simulink model "APF_SoftLanding_Quadrotor"  (R2023a)
settings: Solver=VariableStepAuto  StartTime=0.0  StopTime=120  RelTol=1e-3
values from neighbouring files (symbols this model uses):
  alpha_t = pi/2    (= 1.57079632679)    [Parameters.m]
  d0 = 7    [Parameters.m]
  k1 = 0.1395    [Parameters.m]
  k2 = 0.1784    [Parameters.m]
  k3 = 0.0442    [Parameters.m]
  ka = 0.2    [Parameters.m]
  katt = 10    [Parameters.m]
  kb = 0.6    [Parameters.m]
  kc = 0.4    [Parameters.m]
  krep = 90000    [Parameters.m]
  m = 5    [Parameters.m]
  maxRange = 10    [Parameters.m]
  n = 3    [Parameters.m]
  P_psi_lead = 2    [Parameters.m]
  P_vel_lead = 5    [Parameters.m]
  posHpad = [-25 -25 0]    [Parameters.m]
  Rmin = 0.1    [Parameters.m]
  target = [-25 -25 -5]    [Parameters.m]
  theta_des = pi/4    (= 0.785398163397)    [Parameters.m]
  thresholdLanding = 15    [Parameters.m]
  v_max = 2    [Parameters.m]
  zeta_des = 0    [Parameters.m]
  zGround = -0.15    [Parameters.m]
undefined symbols (not defined in the file or in its folder): Lidar, numobs, obs, platformUAV
libraries: uavsimlib x5, sharedtransform x2, uavalgslib x1, uavutilslib x1
(part 2 of 3)

== matlab function APF_SoftLanding_Quadrotor/MATLAB Function ==
function [V_cmd, yaw_cmd, Stop] = APF_Planner(pos, goal, obs, katt, krep, d0, v_max, numobs)

% =========================================================
% APF Planner for 3D Quadrotor
% pos  : [1x3] UAV position [N E D]
% goal : [1x3] goal position [N E D]
% obs  : [1x3] obstacle position [N E D]
% V_cmd: [1x3] velocity command [VN VE VD]
% =========================================================

% ---------------------------------------------------------
% 1. Initialize outputs with FIXED SIZE
% ---------------------------------------------------------

V_cmd   = zeros(1,3);
yaw_cmd = 0.0;
Stop    = 0.0;
F_att = zeros(1,3);
F_total = zeros(1,3);



% ---------------------------------------------------------
% 2. Force inputs to fixed-size row vectors
% ---------------------------------------------------------

p = zeros(1,3);
g = zeros(1,3);

p(1) = pos(1);
p(2) = pos(2);
p(3) = pos(3);

g(1) = goal(1);
g(2) = goal(2);
g(3) = goal(3);


% Scalar
v_lim = v_max(1);

% Khoảng cách từ UAV đến target
d_goal = g - p;
d_goal_mag = sqrt(d_goal(1)^2 + d_goal(2)^2 + d_goal(3)^2);

% ---------------------------------------------------------
% 3. Attractive force
% ---------------------------------------------------------

    F_att(1) = 2 * katt * d_goal(1);
    F_att(2) = 2 * katt * d_goal(2);
    F_att(3) = 2 * katt * d_goal(3);

% ---------------------------------------------------------
% 4. Repulsive force
% ---------------------------------------------------------



% ---------------------------------------------------------
% 5. Total force
% ---------------------------------------------------------

F_total(1) = F_att(1); 
F_total(2) = F_att(2);
F_total(3) = F_att(3);

F_norm = sqrt(F_total(1)^2 + F_total(2)^2 + F_total(3)^2);


% ---------------------------------------------------------
% 6. Generate velocity command
% ---------------------------------------------------------

if d_goal_mag < 0.15

    V_cmd(1,1) = 0;
    V_cmd(1,2) = 0;
    V_cmd(1,3) = 0;

    Stop = 1.0;

elseif F_norm > 1e-4

    V_cmd(1) = v_lim * F_total(1) / F_norm;
    V_cmd(2) = v_lim * F_total(2) / F_norm;
    V_cmd(3) = v_lim * F_total(3) / F_norm;

else

    V_cmd(1) = 0;
    V_cmd(2) = 0;
    V_cmd(3) = 0;

end

% ---------------------------------------------------------
% 7. Yaw command
% ---------------------------------------------------------

V_horizontal = sqrt(V_cmd(1)^2 + V_cmd(2)^2);

if V_horizontal > 0.05

    yaw_cmd = atan2(V_cmd(2), V_cmd(1));

else

    yaw_cmd = 0.0;

end

end


%% =========================================================================
%% =========================================================================

% function [V_cmd, yaw_cmd, Stop] = APF_Planner(pos, goal, obs, katt, krep, d0, v_max, numobs)
% 
% % =========================================================
% % Improved APF Planner for 3D UAV
% %
% % Coordinate frame: NED
% %
% % FEATURES
% %   1. Attractive force
% %   2. Improved repulsive force for GNRON
% %   3. Local-minimum detection
% %   4. Dynamic tangent escape
% %   5. Forward-looking tangent selection
% %   6. Directional weighting for oscillation suppression
% %   7. Speed scheduling
% %
% % INPUTS
% %   pos     : UAV position        [1x3] [N E D]
% %   goal    : Goal position       [1x3] [N E D]
% %   obs     : Obstacle positions  [Nx3] [N E D]
% %   katt    : Attractive gain
% %   krep    : Repulsive gain
% %   d0      : Obstacle influence distance [m]
% %   v_max   : Maximum velocity [m/s]
% %   numobs  : Number of obstacles
% %
% % OUTPUTS
% %   V_cmd   : Velocity command [1x3] [VN VE VD]
% %   yaw_cmd : Heading command [rad]
% %   Stop    : 1 when goal reached
% %
% % =========================================================
% 
% 
% %% ========================================================
% % 1. INITIALIZATION
% % =========================================================
% 
% V_cmd   = zeros(1,3);
% yaw_cmd = 0.0;
% Stop    = 0.0;
% 
% F_att     = zeros(1,3);
% F_rep     = zeros(1,3);
% F_cmd_raw = zeros(1,3);
% 
% p = zeros(1,3);
% g = zeros(1,3);
% 
% p(1) = pos(1);
% p(2) = pos(2);
% p(3) = pos(3);
% 
% g(1) = goal(1);
% g(2) = goal(2);
% g(3) = goal(3);
% 
% % Đại lượng tránh chia cho 0 
% small_num = 1e-6;
% 
% 
% %% ========================================================
% % 2. PARAMETERS
% % =========================================================
% 
% % Ngưỡng xác định UAV đã tới goal.
% goal_tol = 0.30;          % [m]
% 
% % ---------------------------------------------------------
% % Local minimum detection
% % ---------------------------------------------------------
% 
% % Nếu F_total < F_enter --> Local Minima --> Bật Tangent
% F_enter = 0.10;
% 
% % Nếu F_total > F_exit --> Thoát khỏi Local Minima
% % F_enter < F_total < F_exit --> Vẫn bật Tangent, F_enter < F_exit để tránh Tangent bật tắt liên tục 
% F_exit  = 0.30;
% 
% % Khoảng cách giữa UAV và target phải lớn hơn goal_min_dist thì mới được
% % coi là Local Minima
% goal_min_dist = 0.50;
% 
% 
% % ---------------------------------------------------------
% % Tangential force
% % ---------------------------------------------------------
% 
% % Hệ số độ mạnh của lực tiếp tuyến
% k_tan = 1.0;
% 
% % Number of directions searched on tangent plane (Mặt phẳng tiếp tuyến
% % vuông góc với vector hướng từ Obs ra UAV
% N_tangent = 12;
% 
% % Prediction horizon for tangent evaluation
% N_pred = 3;
% 
% % Prediction distance (Xem UAV sẽ ở đâu)
% look_ahead = 0.25*d0;
% 
% if look_ahead < 0.30
%     look_ahead = 0.30;
% end
% 
% 
% % Tangent candidate cost
% w_goal  = 1.0;
% w_clear = 1.0;
% w_prev  = 0.60;
% 
% 
% % ---------------------------------------------------------
% % Oscillation suppression
% %
% % Δalpha <= pi/6:
% %       m = m'
% %
% % pi/6 < Δalpha <= pi/3:
% %       m > m'
% %
% % Δalpha > pi/3:
% %       m >> m'
% %
% % Numerical values below are implementation choices.
% % ---------------------------------------------------------
% 
% theta_small = pi/6;
% theta_large = pi/3;
% 
% % Small direction change
% m_prev_1 = 0.50;
% m_new_1  = 0.50;
% 
% % Medium direction change
% m_prev_2 = 0.70;
% m_new_2  = 0.30;
% 
% % Large direction change
% m_prev_3 = 0.90;
% m_new_3  = 0.10;
% 
% 
% %% ========================================================
% % 3. PERSISTENT STATES
% % =========================================================
% 
% persistent tangent_active
% persistent tangent_prev
% persistent previous_obs_idx
% 
% persistent prev_move_dir
% persistent prev_dir_valid
% 
% 
% if isempty(tangent_active)
%     tangent_active = false;
% end
% 
% if isempty(tangent_prev)
%     tangent_prev = zeros(1,3);
% end
% 
% if isempty(previous_obs_idx)
%     previous_obs_idx = 0;
% end
% 
% if isempty(prev_move_dir)
%     prev_move_dir = zeros(1,3);
% end
% 
% if isempty(prev_dir_valid)
%     prev_dir_valid = false;
% end
% 
% 
% %% ========================================================
% % 4. NUMBER OF OBSTACLES
% % =========================================================
% 
% Nobs = numobs;
% 
% if Nobs > size(obs,1)
%     Nobs = size(obs,1);
% end
% 
% if Nobs < 0
%     Nobs = 0;
% end
% 
% 
% %% ========================================================
% % 5. GOAL VECTOR
% % =========================================================
% 
% goal_vec = g - p;
% 
% d_goal = sqrt(goal_vec(1)^2 + goal_vec(2)^2 + goal_vec(3)^2);
% 
% 
% %% ========================================================
% % 6. GOAL REACHED
% % =========================================================
% 
% if d_goal <= goal_tol
% 
%     V_cmd   = zeros(1,3);
%     yaw_cmd = 0.0;
%     Stop    = 1.0;
% 
%     % Reset memory
%     tangent_active   = false;
%     tangent_prev     = zeros(1,3);
%     previous_obs_idx = 0;
% 
%     prev_move_dir = zeros(1,3);
%     prev_dir_valid = false;
% 
%     return;
% end
% 
% 
% dir_goal = goal_vec / max(d_goal,small_num);
% 
% 
% %% ========================================================
% % 7. ATTRACTIVE FORCE
% % =========================================================
% %
% % Uatt = katt*d_goal^2
% %
% % Fatt = 2*katt*(goal-pos)
% %
% 
% F_att = 2.0*katt*goal_vec;
% 
% 
% %% ========================================================
% % 8. IMPROVED REPULSIVE FORCE
% %
% % GNRON improvement
% %
% % Frep = Frep1 + Frep2
% % =========================================================
% 
% min_obs_dist = 1e6;
% nearest_idx  = 0;
% 
% 
% for i = 1:Nobs
% 
%     obs_i = zeros(1,3);
% 
%     obs_i(1) = obs(i,1);
%     obs_i(2) = obs(i,2);
%     obs_i(3) = obs(i,3);
% 
% 
%     % Vector obstacle -> UAV
%     obs_vec = p - obs_i;
% 
%     d_obs = sqrt(obs_vec(1)^2 + obs_vec(2)^2 + obs_vec(3)^2);
% 
% 
%     % Nearest obstacle
%     if d_obs < min_obs_dist
%         min_obs_dist = d_obs;
%         nearest_idx  = i;
%     end
% 
% 
%     if d_obs <= d0
% 
%         d_safe = max(d_obs,small_num);
% 
%         dir_away = obs_vec/d_safe;
% 
% 
%         % -------------------------------------------------
%         % Goal-distance weighting
%         %
%         % Approaches zero when UAV approaches goal
%         % -------------------------------------------------
% 
%         exp_goal = exp(-d_goal);
% 
%         weight_rep = 1.0/(1.0 + exp_goal) - 0.5;
% 
% 
%         % -------------------------------------------------
%         % Frep1
%         % -------------------------------------------------
% 
%         coeff1 = 2.0 * krep * (1.0/d_safe - 1.0/d0) * (1.0/(d_safe^2)) * weight_rep;
% 
%         F_rep1 = coeff1 * dir_away;
% 
% 
%         % -------------------------------------------------
%         % Frep2
%         % -------------------------------------------------
% 
%         sigmoid_derivative = exp_goal/((1.0 + exp_goal)^2);
% 
%         coeff2 = krep * (1.0/d_safe - 1.0/d0)^2 * sigmoid_derivative;
% 
%         F_rep2 = coeff2 * dir_goal;
% 
% 
%         F_rep = F_rep + F_rep1 + F_rep2;
% 
%     end
% 
% end
% 
% 
% %% ========================================================
% % 9. NORMAL APF RESULTANT FORCE
% % =========================================================
% 
% F_total = F_att + F_rep;
% 
% F_total_norm = sqrt(F_total(1)^2 + F_total(2)^2 + F_total(3)^2);
% 
% 
% %% ========================================================
% % 10. OBSTACLE NEARBY
% % =========================================================
% 
% obstacle_near = false;
% 
% if (Nobs > 0) && (min_obs_dist < d0)
%     obstacle_near = true;
% end
% 
% 
% %% ========================================================
% % 11. LOCAL MINIMUM DETECTION WITH HYSTERESIS
% % =========================================================
% 
% if ~tangent_active
% 
%     if (F_total_norm < F_enter) && (d_goal > goal_min_dist) && obstacle_near
% 
%         tangent_active = true;
% 
% 
%         % Do not use tangent from unrelated obstacle
%         if nearest_idx ~= previous_obs_idx
%             tangent_prev = zeros(1,3);
%         end
% 
%         previous_obs_idx = nearest_idx;
%     end
% 
% else
% 
%     if (F_total_norm > F_exit) || (~obstacle_near) || (d_goal <= goal_min_dist)
% 
%         tangent_active = false;
% 
%     end
% 
% end
% 
% 
% %% ========================================================
% % 12. DYNAMIC TANGENT ESCAPE
% %
% % Tangent is ONLY added when local minimum is active.
% % =========================================================
% 
% if tangent_active && nearest_idx > 0
% 
%     %% ----------------------------------------------------
%     % 12.1 Nearest obstacle normal
%     % -----------------------------------------------------
% 
%     obs_near = zeros(1,3);
% 
%     obs_near(1) = obs(nearest_idx,1);
%     obs_near(2) = obs(nearest_idx,2);
%     obs_near(3) = obs(nearest_idx,3);
% 
% 
%     normal_vec = p - obs_near;
% 
%     normal_norm = sqrt(normal_vec(1)^2 + normal_vec(2)^2 + normal_vec(3)^2);
% 
% 
%     if normal_norm > small_num
%         n = normal_vec/normal_norm;
%     else
%         n = -dir_goal;
%     end
% 
% 
%     %% ----------------------------------------------------
%     % 12.2 Construct tangent plane basis
%     % -----------------------------------------------------
% 
%     abs_n = abs(n);
% 
%     [~,idx_ref] = min(abs_n);
% 
%     ref = zeros(1,3);
%     ref(idx_ref) = 1.0;
% 
% 
%     e1 = cross(n,ref);
% 
%     e1_norm = sqrt(e1(1)^2 + e1(2)^2 + e1(3)^2);
% 
%     e1 = e1/max(e1_norm,small_num);
% 
% 
%     e2 = cross(n,e1);
% 
%     e2_norm = sqrt(e2(1)^2 + e2(2)^2 + e2(3)^2);
% 
%     e2 = e2/max(e2_norm,small_num);
% 
% 
%     %% ----------------------------------------------------
%     % 12.3 Forward-looking tangent search
%     %
%     % Inspired by paper Eq. (12)-(13)
%     %
%     % Every candidate tangent is predicted several
%     % positions ahead and evaluated by:
%     %
%     %   goal direction
%     %   obstacle clearance
%     %   continuity with previous tangent
%     % -----------------------------------------------------
% 
%     best_score = -1e9;
%     best_tangent = zeros(1,3);
% 
% 
%     tangent_prev_norm = sqrt(tangent_prev(1)^2 + tangent_prev(2)^2 + tangent_prev(3)^2);
% 
% 
%     for k = 1:N_tangent
% 
%         theta = 2.0 * pi * (k-1)/N_tangent;
% 
% 
%         t_candidate = cos(theta) * e1 + sin(theta) * e2;
% 
% 
%         t_norm = sqrt(t_candidate(1)^2 + t_candidate(2)^2 + t_candidate(3)^2);
% 
%         t_candidate = t_candidate/max(t_norm,small_num);
% 
% 
%         % ---------------------------------------------
%         % Goal-direction score
%         % ---------------------------------------------
% 
%         goal_score = dot(t_candidate,dir_goal);
% 
% 
%         % ---------------------------------------------
%         % Previous tangent continuity score
%         % ---------------------------------------------
% 
%         prev_score = 0.0;
% 
%         if tangent_prev_norm > 1e-4
% 
%             prev_tangent_dir = tangent_prev/tangent_prev_norm;
% 
%             prev_score = dot(t_candidate,prev_tangent_dir);
% 
%         end
% 
% 
%         % ---------------------------------------------
%         % Forward-looking clearance
%         % ---------------------------------------------
% 
%         min_pred_dist = 1e6;
% 
% 
%         for h = 1:N_pred
% 
%             pred_ratio = h/N_pred;
% 
%             p_test = p + pred_ratio * look_ahead * t_candidate;
% 
% 
%             for j = 1:Nobs
% 
%                 test_vec = zeros(1,3);
% 
%                 test_vec(1) = p_test(1) - obs(j,1);
% 
%                 test_vec(2) = p_test(2) - obs(j,2);
% 
%                 test_vec(3) = p_test(3) - obs(j,3);
% 
% 
%                 test_dist = sqrt(test_vec(1)^2 + test_vec(2)^2 + test_vec(3)^2);
% 
% 
%                 if test_dist < min_pred_dist
%                     min_pred_dist = test_dist;
%                 end
% 
%             end
% 
%         end
% 
% 
%         clear_score = min_pred_dist/max(d0,small_num);
% 
% 
%         if clear_score > 2.0
%             clear_score = 2.0;
%         end
% 
% 
%         % ---------------------------------------------
%         % Comprehensive score
%         % ---------------------------------------------
% 
%         score = w_goal*goal_score + w_clear*clear_score + w_prev*prev_score;
% 
% 
%         if score > best_score
% 
%             best_score = score;
% 
%             best_tangent = t_candidate;
% 
%         end
% 
%     end
% 
% 
%     % Store tangent for next sample
%     tangent_prev = best_tangent;
% 
% 
%     % Tangential force
%     F_tan = k_tan*best_tangent;
% 
% 
%     % APF + tangent
%     F_cmd_raw = F_total + F_tan;
% 
% 
% else
% 
%     % Normal operation
%     F_cmd_raw = F_total;
% 
% end
% 
% 
% %% ========================================================
% % 13. RAW COMMAND DIRECTION
% % =========================================================
% 
% F_raw_norm = sqrt(F_cmd_raw(1)^2 + F_cmd_raw(2)^2 + F_cmd_raw(3)^2);
% 
% 
% if F_raw_norm > small_num
% 
%     w_new = F_cmd_raw/F_raw_norm;
% 
% else
% 
%     w_new = dir_goal;
% 
% end
% 
% 
% %% ========================================================
% % 14. OSCILLATION SUPPRESSION
% %
% % Based on Eq. (10)-(11) of the paper.
% %
% % Paper:
% %
% % X(n+1) =
% %   X(n) + L*(m*w_n + m'*w_(n+1))
% %
% % Our planner outputs velocity instead of waypoint,
% % therefore:
% %
% % w_cmd =
% %   normalize(m*w_prev + m'*w_new)
% %
% % =========================================================
% 
% move_dir = w_new;
% 
% 
% % Apply directional continuity mainly near obstacles.
% if obstacle_near && prev_dir_valid
% 
%     % -----------------------------------------------------
%     % Angle between previous and current directions
%     % -----------------------------------------------------
% 
%     cos_alpha = dot(prev_move_dir,w_new);
% 
% 
%     % Numerical clamp
%     if cos_alpha > 1.0
%         cos_alpha = 1.0;
%     elseif cos_alpha < -1.0
%         cos_alpha = -1.0;
%     end
% 
% 
%     delta_alpha = acos(cos_alpha);
% 
% 
%     % -----------------------------------------------------
%     % Direction weighting according to paper Eq. (11)
%     % -----------------------------------------------------
% 
%     if delta_alpha <= theta_small
% 
%         % m = m'
%         m_prev = m_prev_1;
%         m_new  = m_new_1;
% 
% 
%     elseif delta_alpha <= theta_large
% 
%         % m > m'
%         m_prev = m_prev_2;
%         m_new  = m_new_2;
% 
% 
%     else
% 
%         % m >> m'
%         m_prev = m_prev_3;
%         m_new  = m_new_3;
% 
%     end
% 
% 
%     % -----------------------------------------------------
%     % Eq. (10)-style weighted direction
%     % -----------------------------------------------------
% 
%     w_weighted = m_prev*prev_move_dir + m_new*w_new;
% 
% 
%     w_weighted_norm = sqrt(w_weighted(1)^2 + w_weighted(2)^2 + w_weighted(3)^2);
% 
% 
%     if w_weighted_norm > small_num
% 
%         move_dir = w_weighted/w_weighted_norm;
% 
%     else
% 
%         move_dir = w_new;
% 
%     end
% 
% end
% 
% 
% % ---------------------------------------------------------
% % Save actual direction used
% % ---------------------------------------------------------
% 
% prev_move_dir = move_dir;
% prev_dir_valid = true;
% 
% 
% %% ========================================================
% % 15. SPEED SCHEDULING
% % =========================================================
% 
% % Slow near goal
% goal_speed_factor = d_goal/max(d0,small_num);
% 
% 
% if goal_speed_factor > 1.0
%     goal_speed_factor = 1.0;
% elseif goal_speed_factor < 0.15
%     goal_speed_factor = 0.15;
% end
% 
% 
% % Slow near obstacles
% obs_speed_factor = 1.0;
% 
% 
% if obstacle_near
% 
%     obs_speed_factor = min_obs_dist/max(d0,small_num);
% 
% 
%     if obs_speed_factor < 0.25
%         obs_speed_factor = 0.25;
%     elseif obs_speed_factor > 1.0
%         obs_speed_factor = 1.0;
%     end
% 
% end
% 
% 
% v_cmd_mag = v_max * goal_speed_factor * obs_speed_factor;
% 
% 
% % Do not become too slow while escaping local minimum
% if tangent_active
% 
%     v_escape_min = 0.35*v_max;
% 
%     if v_cmd_mag < v_escape_min
%         v_cmd_mag = v_escape_min;
%     end
% 
% end
% 
% 
% %% ========================================================
% % 16. VELOCITY COMMAND
% % =========================================================
% 
% V_cmd = v_cmd_mag * move_dir;
% 
% 
% %% ========================================================
% % 17. YAW COMMAND
% % =========================================================
% 
% horizontal_speed = sqrt(V_cmd(1)^2 + V_cmd(2)^2);
% 
% 
% if horizontal_speed > small_num
% 
%     yaw_cmd = atan2(V_cmd(2),V_cmd(1));
% 
% else
% 
%     yaw_cmd = 0.0;
% 
% end
% 
% 
% Stop = 0.0;
% 
% end

%% ============================================================================
%% ===============================================================================

% function [V_cmd, yaw_cmd, Stop] = APF_Planner( ...
%     pos, goal, obs, katt, krep, d0, v_max, numobs)
% 
% % =========================================================
% % Improved APF Planner for 3D UAV
% %
% % Coordinate frame: NED
% %
% % Features:
% %   1. Attractive force
% %   2. Improved repulsive force for GNRON
% %   3. Local-minimum detection using resultant force
% %   4. Dynamic optimal tangential force
% %   5. Tangent hysteresis
% %   6. Tangent direction memory
% %   7. Speed scheduling
% %
% % INPUTS:
% %   pos     : UAV position        [1x3] [N E D]
% %   goal    : Goal position       [1x3] [N E D]
% %   obs     : Obstacle positions  [Nx3] [N E D]
% %   katt    : Attractive gain
% %   krep    : Repulsive gain
% %   d0      : Obstacle influence distance [m]
% %   v_max   : Maximum velocity [m/s]
% %   numobs  : Number of obstacles
% %
% % OUTPUTS:
% %   V_cmd   : Velocity command [1x3] [VN VE VD]
% %   yaw_cmd : Heading command [rad]
% %   Stop    : 1 when goal reached
% %
% % =========================================================
% 
% 
% %% ========================================================
% % 1. FIXED-SIZE INITIALIZATION
% % =========================================================
% 
% V_cmd   = zeros(1,3);
% yaw_cmd = 0.0;
% Stop    = 0.0;
% 
% F_att   = zeros(1,3);
% F_rep   = zeros(1,3);
% F_total = zeros(1,3);
% F_cmd   = zeros(1,3);
% 
% p = zeros(1,3);
% g = zeros(1,3);
% 
% p(1) = pos(1);
% p(2) = pos(2);
% p(3) = pos(3);
% 
% g(1) = goal(1);
% g(2) = goal(2);
% g(3) = goal(3);
% 
% small_num = 1e-6;
% 
% 
% %% ========================================================
% % 2. PARAMETERS
% % =========================================================
% 
% % Goal tolerance
% goal_tol = 0.30;          % [m]
% 
% % ---------------------------------------------------------
% % Local minimum detection
% % ---------------------------------------------------------
% %
% % Tangent is activated when:
% %
% %       |F_total| < F_enter
% %
% % and deactivated only when:
% %
% %       |F_total| > F_exit
% %
% % F_exit > F_enter creates hysteresis.
% %
% % IMPORTANT:
% % These values must be tuned according to katt/krep.
% % ---------------------------------------------------------
% 
% F_enter = 0.10;
% F_exit  = 0.30;
% 
% % UAV must still be sufficiently far from goal
% goal_min_dist = 0.50;     % [m]
% 
% 
% % ---------------------------------------------------------
% % Tangential force
% % ---------------------------------------------------------
% 
% k_tan = 1.0;
% 
% % Number of tangent candidate directions
% %
% % 12 -> every 30 degrees in tangent plane
% N_tangent = 12;
% 
% % Look-ahead distance used to evaluate tangent direction
% look_ahead = 0.25 * d0;
% 
% if look_ahead < 0.30
%     look_ahead = 0.30;
% end
% 
% % Cost-function weights
% w_goal  = 1.0;
% w_clear = 1.0;
% w_prev  = 0.6;
% 
% 
% %% ========================================================
% % 3. PERSISTENT STATES FOR TANGENT MODE
% % =========================================================
% 
% persistent tangent_active
% persistent tangent_prev
% persistent previous_obs_idx
% 
% if isempty(tangent_active)
%     tangent_active = false;
% end
% 
% if isempty(tangent_prev)
%     tangent_prev = zeros(1,3);
% end
% 
% if isempty(previous_obs_idx)
%     previous_obs_idx = 0;
% end
% 
% 
% %% ========================================================
% % 4. NUMBER OF OBSTACLES
% % =========================================================
% 
% Nobs = numobs;
% 
% if Nobs > size(obs,1)
%     Nobs = size(obs,1);
% end
% 
% if Nobs < 0
%     Nobs = 0;
% end
% 
% 
% %% ========================================================
% % 5. VECTOR TO GOAL
% % =========================================================
% 
% goal_vec = g - p;
% 
% d_goal = sqrt( ...
%     goal_vec(1)^2 + ...
%     goal_vec(2)^2 + ...
%     goal_vec(3)^2);
% 
% 
% %% ========================================================
% % 6. GOAL REACHED
% % =========================================================
% 
% if d_goal <= goal_tol
% 
%     V_cmd   = zeros(1,3);
%     yaw_cmd = 0.0;
%     Stop    = 1.0;
% 
%     % Reset tangent state
%     tangent_active   = false;
%     tangent_prev     = zeros(1,3);
%     previous_obs_idx = 0;
% 
%     return;
% 
% end
% 
% 
% % Unit vector toward goal
% dir_goal = goal_vec / max(d_goal, small_num);
% 
% 
% %% ========================================================
% % 7. ATTRACTIVE FORCE
% %
% % U_att = katt * d_goal^2
% %
% % F_att = 2*katt*(goal-pos)
% % =========================================================
% 
% F_att = 2.0 * katt * goal_vec;
% 
% 
% %% ========================================================
% % 8. IMPROVED REPULSIVE FORCE FOR GNRON
% % =========================================================
% 
% min_obs_dist = 1e6;
% nearest_idx  = 0;
% 
% 
% for i = 1:Nobs
% 
%     obs_i = zeros(1,3);
% 
%     obs_i(1) = obs(i,1);
%     obs_i(2) = obs(i,2);
%     obs_i(3) = obs(i,3);
% 
% 
%     % -----------------------------------------------------
%     % Vector from obstacle toward UAV
%     % -----------------------------------------------------
% 
%     obs_vec = p - obs_i;
% 
%     d_obs = sqrt( ...
%         obs_vec(1)^2 + ...
%         obs_vec(2)^2 + ...
%         obs_vec(3)^2);
% 
% 
%     % Find nearest obstacle
%     if d_obs < min_obs_dist
% 
%         min_obs_dist = d_obs;
%         nearest_idx  = i;
% 
%     end
% 
% 
%     % -----------------------------------------------------
%     % Only active inside obstacle influence distance
%     % -----------------------------------------------------
% 
%     if d_obs <= d0
% 
%         d_safe = max(d_obs, small_num);
% 
% 
%         % Unit direction away from obstacle
%         dir_away = obs_vec / d_safe;
% 
% 
%         % =================================================
%         % Goal-distance weighting
%         %
%         % Positive version of the weighting term is used
%         % here so that Frep1 points AWAY from obstacle.
%         %
%         % As d_goal -> 0:
%         %
%         % weight_rep -> 0
%         %
%         % therefore obstacle repulsion weakens near goal.
%         % =================================================
% 
%         exp_goal = exp(-d_goal);
% 
%         weight_rep = ...
%             1.0 / (1.0 + exp_goal) - 0.5;
% 
% 
%         % =================================================
%         % Frep1
%         % Main obstacle repulsive component
%         % =================================================
% 
%         coeff1 = ...
%             2.0 * krep ...
%             * (1.0/d_safe - 1.0/d0) ...
%             * (1.0/(d_safe^2)) ...
%             * weight_rep;
% 
%         F_rep1 = coeff1 * dir_away;
% 
% 
%         % =================================================
%         % Frep2
%         % Goal-oriented component
%         % =================================================
% 
%         sigmoid_derivative = ...
%             exp_goal / ((1.0 + exp_goal)^2);
% 
% 
%         coeff2 = ...
%             krep ...
%             * (1.0/d_safe - 1.0/d0)^2 ...
%             * sigmoid_derivative;
% 
% 
%         F_rep2 = coeff2 * dir_goal;
% 
% 
%         % =================================================
%         % Total obstacle contribution
%         % =================================================
% 
%         F_rep = F_rep + F_rep1 + F_rep2;
% 
%     end
% 
% end
% 
% 
% %% ========================================================
% % 9. NORMAL APF RESULTANT FORCE
% % =========================================================
% 
% F_total = F_att + F_rep;
% 
% F_norm = sqrt( ...
%     F_total(1)^2 + ...
%     F_total(2)^2 + ...
%     F_total(3)^2);
% 
% 
% %% ========================================================
% % 10. LOCAL MINIMUM / TANGENT ACTIVATION
% % =========================================================
% 
% % Tangent only allowed if an obstacle is actually nearby
% obstacle_near = false;
% 
% if (Nobs > 0) && (min_obs_dist < d0)
%     obstacle_near = true;
% end
% 
% 
% % ---------------------------------------------------------
% % Enter tangent mode
% % ---------------------------------------------------------
% 
% if ~tangent_active
% 
%     if (F_norm < F_enter) && ...
%        (d_goal > goal_min_dist) && ...
%        obstacle_near
% 
%         tangent_active = true;
% 
%         % New obstacle -> do not inherit tangent direction
%         % from an unrelated previous obstacle
%         if nearest_idx ~= previous_obs_idx
%             tangent_prev = zeros(1,3);
%         end
% 
%         previous_obs_idx = nearest_idx;
% 
%     end
% 
% else
% 
%     % -----------------------------------------------------
%     % Exit tangent mode
%     %
%     % Hysteresis:
%     %
%     % F_exit > F_enter
%     % -----------------------------------------------------
% 
%     if (F_norm > F_exit) || ...
%        (~obstacle_near) || ...
%        (d_goal <= goal_min_dist)
% 
%         tangent_active = false;
% 
%     end
% 
% end
% 
% 
% %% ========================================================
% % 11. DYNAMIC OPTIMAL TANGENT
% % =========================================================
% 
% if tangent_active && nearest_idx > 0
% 
%     % -----------------------------------------------------
%     % Nearest obstacle
%     % -----------------------------------------------------
% 
%     obs_near = zeros(1,3);
% 
%     obs_near(1) = obs(nearest_idx,1);
%     obs_near(2) = obs(nearest_idx,2);
%     obs_near(3) = obs(nearest_idx,3);
% 
% 
%     % -----------------------------------------------------
%     % Normal vector of obstacle surface
%     %
%     % n points:
%     %
%     % obstacle ---> UAV
%     % -----------------------------------------------------
% 
%     normal_vec = p - obs_near;
% 
%     normal_norm = sqrt( ...
%         normal_vec(1)^2 + ...
%         normal_vec(2)^2 + ...
%         normal_vec(3)^2);
% 
% 
%     if normal_norm > small_num
% 
%         n = normal_vec / normal_norm;
% 
%     else
% 
%         % Extremely unlikely case:
%         % UAV exactly at obstacle center
%         n = -dir_goal;
% 
%     end
% 
% 
%     % =====================================================
%     % 11.1 CREATE ORTHONORMAL BASIS ON TANGENT PLANE
%     %
%     % Choose reference axis least parallel to n.
%     %
%     % This axis is ONLY used to construct the tangent plane.
%     % Final tangent direction is optimized over 360 degrees.
%     % =====================================================
% 
%     abs_n = abs(n);
% 
%     [~, idx_ref] = min(abs_n);
% 
%     ref = zeros(1,3);
%     ref(idx_ref) = 1.0;
% 
% 
%     % First tangent basis vector
%     e1 = cross(n, ref);
% 
%     e1_norm = sqrt( ...
%         e1(1)^2 + ...
%         e1(2)^2 + ...
%         e1(3)^2);
% 
%     e1 = e1 / max(e1_norm, small_num);
% 
% 
%     % Second tangent basis vector
%     e2 = cross(n, e1);
% 
%     e2_norm = sqrt( ...
%         e2(1)^2 + ...
%         e2(2)^2 + ...
%         e2(3)^2);
% 
%     e2 = e2 / max(e2_norm, small_num);
% 
% 
%     % =====================================================
%     % 11.2 SEARCH BEST TANGENT DIRECTION
%     % =====================================================
% 
%     best_score = -1e9;
% 
%     best_tangent = zeros(1,3);
% 
% 
%     tangent_prev_norm = sqrt( ...
%         tangent_prev(1)^2 + ...
%         tangent_prev(2)^2 + ...
%         tangent_prev(3)^2);
% 
% 
%     for k = 1:N_tangent
% 
%         % ---------------------------------------------
%         % Candidate tangent direction
%         %
%         % Covers complete 360 deg tangent plane
%         % ---------------------------------------------
% 
%         theta = ...
%             2.0*pi*(k-1)/N_tangent;
% 
% 
%         t_candidate = ...
%             cos(theta)*e1 + ...
%             sin(theta)*e2;
% 
% 
%         % Already unit length theoretically,
%         % but normalize for numerical safety
%         t_norm = sqrt( ...
%             t_candidate(1)^2 + ...
%             t_candidate(2)^2 + ...
%             t_candidate(3)^2);
% 
%         t_candidate = ...
%             t_candidate / max(t_norm, small_num);
% 
% 
%         % =================================================
%         % A. GOAL PROGRESS SCORE
%         %
%         % +1 : directly toward goal
%         %  0 : perpendicular
%         % -1 : away from goal
%         % =================================================
% 
%         goal_score = ...
%             dot(t_candidate, dir_goal);
% 
% 
%         % =================================================
%         % B. PREVIOUS DIRECTION SCORE
%         %
%         % Reduces left-right switching.
%         % =================================================
% 
%         prev_score = 0.0;
% 
%         if tangent_prev_norm > 1e-4
% 
%             prev_dir = ...
%                 tangent_prev / tangent_prev_norm;
% 
%             prev_score = ...
%                 dot(t_candidate, prev_dir);
% 
%         end
% 
% 
%         % =================================================
%         % C. OBSTACLE CLEARANCE SCORE
%         %
%         % Predict position after one look-ahead step.
%         % =================================================
% 
%         p_test = ...
%             p + look_ahead*t_candidate;
% 
% 
%         min_test_dist = 1e6;
% 
% 
%         for j = 1:Nobs
% 
%             test_vec = zeros(1,3);
% 
%             test_vec(1) = ...
%                 p_test(1) - obs(j,1);
% 
%             test_vec(2) = ...
%                 p_test(2) - obs(j,2);
% 
%             test_vec(3) = ...
%                 p_test(3) - obs(j,3);
% 
% 
%             test_dist = sqrt( ...
%                 test_vec(1)^2 + ...
%                 test_vec(2)^2 + ...
%                 test_vec(3)^2);
% 
% 
%             if test_dist < min_test_dist
%                 min_test_dist = test_dist;
%             end
% 
%         end
% 
% 
%         % Normalize clearance approximately with d0
%         clear_score = min_test_dist / max(d0,small_num);
% 
%         % Limit excessive influence
%         if clear_score > 2.0
%             clear_score = 2.0;
%         end
% 
% 
%         % =================================================
%         % D. TOTAL SCORE
%         % =================================================
% 
%         score = ...
%             w_goal  * goal_score  + ...
%             w_clear * clear_score + ...
%             w_prev  * prev_score;
% 
% 
%         % =================================================
%         % Select best tangent
%         % =================================================
% 
%         if score > best_score
% 
%             best_score   = score;
%             best_tangent = t_candidate;
% 
%         end
% 
%     end
% 
% 
%     % -----------------------------------------------------
%     % Save tangent direction for next sample
%     % -----------------------------------------------------
% 
%     tangent_prev = best_tangent;
% 
% 
%     % =====================================================
%     % 11.3 TANGENTIAL FORCE
%     % =====================================================
% 
%     F_tan = k_tan * best_tangent;
% 
% 
%     % =====================================================
%     % APF + tangent
%     % =====================================================
% 
%     F_cmd = F_total + F_tan;
% 
% 
% else
% 
%     % =====================================================
%     % Normal APF
%     %
%     % Tangent does NOT affect UAV here.
%     % =====================================================
% 
%     F_cmd = F_total;
% 
% end
% 
% 
% %% ========================================================
% % 12. COMMAND DIRECTION
% % =========================================================
% 
% F_cmd_norm = sqrt( ...
%     F_cmd(1)^2 + ...
%     F_cmd(2)^2 + ...
%     F_cmd(3)^2);
% 
% 
% if F_cmd_norm > small_num
% 
%     move_dir = F_cmd / F_cmd_norm;
% 
% else
% 
%     % Safety fallback
%     move_dir = dir_goal;
% 
% end
% 
% 
% %% ========================================================
% % 13. SPEED SCHEDULING
% % =========================================================
% 
% % ---------------------------------------------------------
% % Reduce speed when approaching goal
% % ---------------------------------------------------------
% 
% goal_speed_factor = d_goal / max(d0,small_num);
% 
% if goal_speed_factor > 1.0
%     goal_speed_factor = 1.0;
% end
% 
% if goal_speed_factor < 0.15
%     goal_speed_factor = 0.15;
% end
% 
% 
% % ---------------------------------------------------------
% % Reduce speed near obstacles
% % ---------------------------------------------------------
% 
% obs_speed_factor = 1.0;
% 
% if obstacle_near
% 
%     obs_speed_factor = ...
%         min_obs_dist / max(d0,small_num);
% 
%     if obs_speed_factor < 0.25
%         obs_speed_factor = 0.25;
%     end
% 
%     if obs_speed_factor > 1.0
%         obs_speed_factor = 1.0;
%     end
% 
% end
% 
% 
% % ---------------------------------------------------------
% % Final velocity magnitude
% % ---------------------------------------------------------
% 
% v_cmd_mag = ...
%     v_max ...
%     * goal_speed_factor ...
%     * obs_speed_factor;
% 
% 
% % ---------------------------------------------------------
% % While escaping local minimum, do not allow UAV
% % to become excessively slow.
% % ---------------------------------------------------------
% 
% if tangent_active
% 
%     min_escape_speed = 0.35*v_max;
% 
%     if v_cmd_mag < min_escape_speed
%         v_cmd_mag = min_escape_speed;
%     end
% 
% end
% 
% 
% %% ========================================================
% % 14. VELOCITY COMMAND
% % =========================================================
% 
% V_cmd = v_cmd_mag * move_dir;
% 
% 
% %% ========================================================
% % 15. YAW COMMAND
% %
% % NED:
% %
% % yaw = atan2(East, North)
% % =========================================================
% 
% horizontal_speed = sqrt( ...
%     V_cmd(1)^2 + ...
%     V_cmd(2)^2);
% 
% 
% if horizontal_speed > small_num
% 
%     yaw_cmd = ...
%         atan2(V_cmd(2), V_cmd(1));
% 
% else
% 
%     yaw_cmd = 0.0;
% 
% end
% 
% 
% Stop = 0.0;
% 
% end

== matlab function APF_SoftLanding_Quadrotor/Subsystem/obstacleDetection ==
function [obstaclePos, obstacleClosest, obstacleSize, numObstacles] = ...
    obstacleDetection(pointsNED, uavPosNED)

%% =========================================================
%  OBSTACLE DETECTION FROM LiDAR POINT CLOUD
%
%  Module 3:
%       ROI filtering + Ground removal
%
%  Module 4:
%       Euclidean clustering
%
%  Module 5:
%       Obstacle position + closest point + size
%
%  INPUT:
%       pointsNED    : Nx3 LiDAR point cloud in NED frame
%       uavPosNED    : 1x3 UAV position [N E D]
%
%  OUTPUT:
%       obstaclePos      : MaxObs x 3 obstacle centroid
%       obstacleClosest  : MaxObs x 3 closest point
%       obstacleSize     : MaxObs x 3 bounding box size
%       numObstacles     : number of detected obstacles
%% =========================================================


%% ===================== PARAMETERS =========================

% Maximum detection range
MAX_RANGE = 15.0;       % [m]

% ROI in NED frame relative to UAV
N_FORWARD  = 15.0;      % [m]
N_BACKWARD = 3.0;       % [m]

E_LEFT  = 8.0;           % [m]
E_RIGHT = 8.0;           % [m]

D_UP   = -8.0;           % [m]
D_DOWN = 8.0;            % [m]

% Ground height relative to UAV
GROUND_MARGIN = 0.5;     % [m]

% Clustering distance
CLUSTER_DISTANCE = 0.7;  % [m]

% Minimum number of points in a cluster
MIN_POINTS = 20;

% Maximum number of obstacles returned
MAX_OBSTACLES = 10;


%% ===================== INITIALIZATION =====================

obstaclePos     = zeros(MAX_OBSTACLES,3);
obstacleClosest = zeros(MAX_OBSTACLES,3);
obstacleSize    = zeros(MAX_OBSTACLES,3);

numObstacles = 0;


%% ===================== CHECK INPUT =========================

if isempty(pointsNED)
    return;
end

% Force Nx3
pointsNED = reshape(pointsNED,[],3);

% Force UAV position to 1x3
uavPosNED = reshape(uavPosNED,1,3);


%% ===================== REMOVE NaN / Inf ===================

valid = all(isfinite(pointsNED),2);

pointsNED = pointsNED(valid,:);

if isempty(pointsNED)
    return;
end


%% ===================== MODULE 3 ===========================
%                    ROI FILTERING
%
% Convert absolute NED coordinates into coordinates
% relative to UAV.

relativePoints = pointsNED - uavPosNED;


% NED:
%
% N = North
% E = East
% D = Down
%
% Forward direction is assumed to be +N.

idxROI = ...
    relativePoints(:,1) >= -N_BACKWARD & ...
    relativePoints(:,1) <=  N_FORWARD  & ...
    relativePoints(:,2) >= -E_LEFT     & ...
    relativePoints(:,2) <=  E_RIGHT    & ...
    relativePoints(:,3) >=  D_UP       & ...
    relativePoints(:,3) <=  D_DOWN;


pointsNED = pointsNED(idxROI,:);

relativePoints = relativePoints(idxROI,:);


if isempty(pointsNED)
    return;
end


%% ===================== RANGE FILTER ========================

distance = sqrt( ...
    relativePoints(:,1).^2 + ...
    relativePoints(:,2).^2 + ...
    relativePoints(:,3).^2 );


idxRange = distance <= MAX_RANGE;

pointsNED = pointsNED(idxRange,:);
relativePoints = relativePoints(idxRange,:);


if isempty(pointsNED)
    return;
end


%% ===================== GROUND REMOVAL ======================
%
% NED convention:
%
%       D increases downward
%
% Therefore ground is located at larger D.
%
% We estimate ground approximately from the lowest
% detected points.
%

groundLevel = max(pointsNED(:,3));

idxGround = pointsNED(:,3) < ...
            groundLevel - GROUND_MARGIN;

pointsNED = pointsNED(idxGround,:);


if isempty(pointsNED)
    return;
end


%% ===================== MODULE 4 ============================
%                    CLUSTERING
%
% Simple Euclidean clustering.
%
% Two points belong to the same cluster if their
% distance is smaller than CLUSTER_DISTANCE.


N = size(pointsNED,1);

labels = zeros(N,1);

clusterID = 0;


for i = 1:N

    if labels(i) ~= 0
        continue;
    end

    % Start new cluster
    clusterID = clusterID + 1;

    labels(i) = clusterID;

    changed = true;

    while changed

        changed = false;

        clusterPoints = find(labels == clusterID);

        for j = 1:N

            if labels(j) ~= 0
                continue;
            end

            % Check distance to all current cluster points
            for k = 1:length(clusterPoints)

                p1 = pointsNED(clusterPoints(k),:);
                p2 = pointsNED(j,:);

                d = sqrt(sum((p1-p2).^2));

                if d <= CLUSTER_DISTANCE

                    labels(j) = clusterID;

                    changed = true;

                    break;
                end

            end

        end

    end

end


%% ===================== MODULE 5 ============================
%                OBSTACLE EXTRACTION
%
% For every cluster:
%
% 1. Remove small clusters
% 2. Calculate centroid
% 3. Find closest point to UAV
% 4. Calculate bounding box


for k = 1:clusterID

    idx = labels == k;

    cluster = pointsNED(idx,:);

    numPoints = size(cluster,1);


    %% Remove small cluster

    if numPoints < MIN_POINTS
        continue;
    end


    %% Check maximum number of obstacles

    if numObstacles >= MAX_OBSTACLES
        break;
    end


    %% Increment obstacle count

    numObstacles = numObstacles + 1;


    %% Centroid

    centroid = mean(cluster,1);

    obstaclePos(numObstacles,:) = centroid;


    %% Closest point to UAV

    relativeCluster = cluster - uavPosNED;

    distances = sqrt(sum(relativeCluster.^2,2));

    [~,idxMin] = min(distances);

    obstacleClosest(numObstacles,:) = ...
        cluster(idxMin,:);


    %% Bounding box

    minPoint = min(cluster,[],1);
    maxPoint = max(cluster,[],1);

    obstacleSize(numObstacles,:) = ...
        maxPoint - minPoint;

end

end

== matlab function APF_SoftLanding_Quadrotor/Subsystem/detectObstaclesNED ==
function [numObstacles, obstacles, rSafe] = detectObstaclesNED(ptsNED, zGround, maxRange)
% DETECTOBSTACLESNED Trích xuất vật cản từ đám mây điểm hệ NED
%
% Đầu vào:
%   ptsNED   : Ma trận Nx3 [X, Y, Z] chứa tọa độ đám mây điểm (hệ NED)
%   zGround  : Giới hạn độ cao mặt đất (m) (NED: Z hướng xuống, vd: sàn ở 0 thì zGround = -0.15)
%   maxRange : Bán kính quan sát tối đa tính từ gốc tọa độ (m), mặc định 10m
%
% Đầu ra:
%   numObstacles : Tổng số lượng vật cản phát hiện được
%   obstacles    : Ma trận Kx7 chứa thông tin K vật cản:
%                  [Xc, Yc, Zc, dx, dy, dz, r_safe]
%                  - (Xc, Yc, Zc): Tọa độ tâm hình học trong hệ NED
%                  - (dx, dy, dz): Kích thước bao (dài, rộng, cao)
%                  - r_safe      : Bán kính bao hình cầu (bounding sphere)

    if nargin < 3, maxRange = 10; end
    if nargin < 2, zGround = -0.15; end

    % Khởi tạo đầu ra rỗng
    numObstacles = 0;
    obstacles = zeros(0, 7);

    if isempty(ptsNED)
        return;
    end

    % 1. Lọc điểm: Loại bỏ sàn đất và các điểm nằm ngoài bán kính quan sát
    horizDist = hypot(ptsNED(:, 1), ptsNED(:, 2));
    validMask = (ptsNED(:, 3) < zGround) & (horizDist <= maxRange);
    filteredPts = ptsNED(validMask, :);

    if size(filteredPts, 1) < 15
        return; % Quá ít điểm, xem như không có vật cản thực thể
    end

    % 2. Giảm mật độ điểm (Voxel Grid) để thuật toán chạy thời gian thực
    ptCloudObj = pointCloud(filteredPts);
    gridStep = 0.08; % Độ phân giải voxel: 8 cm
    downsampledCloud = pcdownsample(ptCloudObj, 'gridAverage', gridStep);
    ptsProcessing = downsampledCloud.Location;

    % 3. Phân cụm điểm (DBSCAN)
    epsilon = 0.35; % Khoảng cách liên kết tối đa giữa 2 điểm cùng một vật thể (m)
    minPoints = 6;  % Số điểm tối thiểu để tạo thành một vật thể hợp lệ
    labels = dbscan(ptsProcessing, epsilon, minPoints);

    uniqueClusters = unique(labels);
    uniqueClusters(uniqueClusters <= 0) = []; % Loại bỏ nhãn nhiễu (-1)

    numObstacles = length(uniqueClusters);
    if numObstacles == 0
        return;
    end

    % 4. Tính toán tọa độ tâm và kích thước từng vật cản
    obstacles = zeros(numObstacles, 7);

    for k = 1:numObstacles
        cId = uniqueClusters(k);
        cPoints = ptsProcessing(labels == cId, :);

        % Tọa độ tâm hình học (Xc, Yc, Zc)
        center = mean(cPoints, 1);

        % Kích thước hộp bao (dx, dy, dz)
        minBounds = min(cPoints, [], 1);
        maxBounds = max(cPoints, [], 1);
        dimensions = maxBounds - minBounds;

        % Bán kính bao hình cầu phục vụ tránh va chạm
        distsToCenter = sqrt(sum((cPoints - center).^2, 2));
        rSafe = max(distsToCenter);

        obstacles(k, :) = center;
    end
end
